simulink subsystem "Follow_Gap_Compute"  (R2023b)
settings: Solver=VariableStepAuto  StartTime=0.0  StopTime=10.0  RelTol=1e-3
libraries: robotlib x2
settings Model: Creator=pmodi  LastModifiedBy=abbas

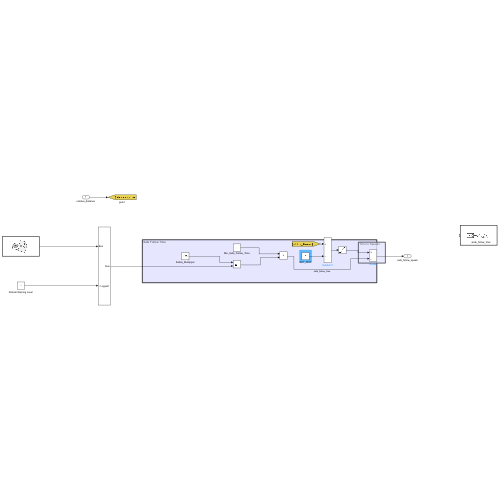
[thumbnail: Simulink's stored preview of the top-level diagram]
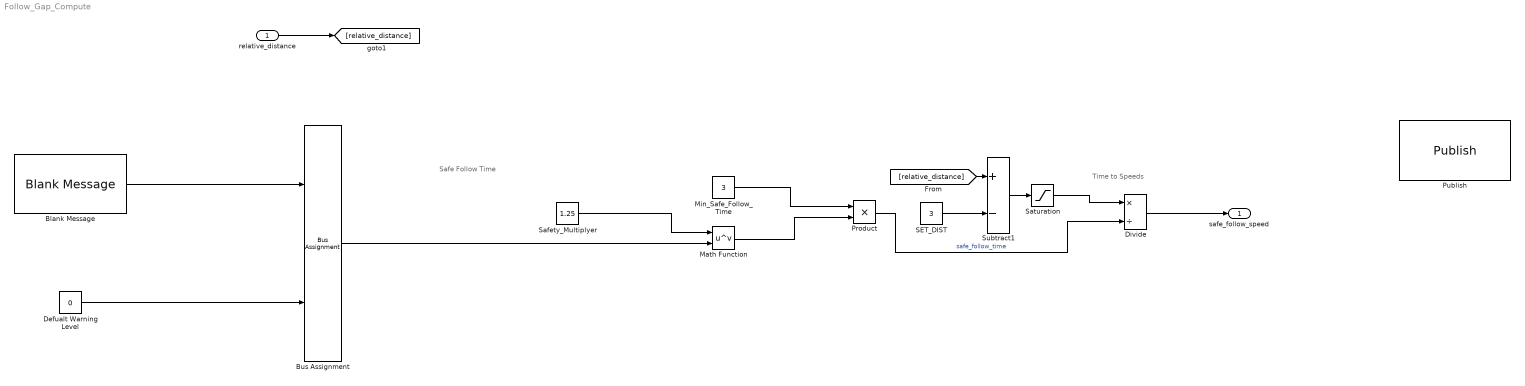
== system Follow_Gap_Compute ==
  note: Safe Follow Time
  note: Time to Speeds
  relative_distance : Inport
  Blank Message : robotlib/Blank Message  messageClass=Message  entityType=geometry_msgs/Point  messageType=geometry_msgs/Point  SampleTime=inf  legacyBusStruct=off
  Bus Assignment : BusAssignment  AssignedSignals=signal1
  Defualt Warning Level : Constant  Value=0
  Divide : Product  Inputs=*/
  Math Function : Math  Operator=pow
  Min_Safe_Follow_Time : Constant  Value=3
  Product : Product
  Publish : robotlib/Publish  topicSource=Specify your own  topic=/safe_follow_time  messageType=geometry_msgs/Point  legacyBusStruct=off  messageQueueLength=1
  SET_DIST : Constant  Value=3
  Safety_Multiplyer : Constant  Value=1.25
  Saturation : Saturate  UpperLimit=inf  LowerLimit=0
  Subtract1 : Sum  Inputs=+-
  safe_follow_speed : Outport
  wires:
  Min_Safe_Follow_Time/1 -> Product/1
  Safety_Multiplyer/1 -> Math Function/1
  Bus Assignment/1 -> Math Function/2
  Math Function/1 -> Product/2
  Blank Message/1 -> Bus Assignment/1
  Defualt Warning Level/1 -> Bus Assignment/2
  Divide/1 -> safe_follow_speed/1
  Saturation/1 -> Divide/1
  Subtract1/1 -> Saturation/1
  Product/1 -> Divide/2  "safe_follow_time"
  [relative_distance] -> Subtract1/1
  SET_DIST/1 -> Subtract1/2
  relative_distance/1 -> [relative_distance]
